simulink model "Tank_test_init_sim_2017b"  (R2017b)
settings: Solver=FixedStepAuto  StartTime=0.0  StopTime=Endtime  FixedStep=Ts_sys  RelTol=1e-3
StopFcn:
  | %ファイル出力
  | %======================== 全体 =================================
  | time = Tank_IOdata_All.time;
  | %状態変数
  | Pipe_Temp1 = Tank_IOdata_All.signals.values(:, 1);
  | Pipe_Temp2 = Tank_IOdata_All.signals.values(:, 2);
  | Pipe_Temp3 = Tank_IOdata_All.signals.values(:, 3);
  | Tank1_Height = Tank_IOdata_All.signals.values(:, 4);
  | Tank2_Height = Tank_IOdata_All.signals.values(:, 5);
  | Cold_Flow = Tank_IOdata_All.signals.values(:, 6);
  | Hot_Flow = Tank_IOdata_All.signals.values(:, 7);
  | Discharge_Flow1 =  Tank_IOdata_All.signals.values(:, 8);
  | Discharge_Flow2 =  Tank_IOdata_All.signals.values(:, 9);
  | %入力
  | u_Cold =  Tank_IOdata_All.signals.values(:, 10);
  | u_Hot =  Tank_IOdata_All.signals.values(:, 11);
  | u_Heater =  Tank_IOdata_All.signals.values(:, 12);
  | u_Valve =  Tank_IOdata_All.signals.values(:, 13);
  | 
  | %ファイル出力
  | filename = 'Tank_test';
  | %matファイル出力
  | save([filename, '.mat']);
  | %csv出力
  | fid = fopen([filename, '.csv'],'w');
  | fprintf(fid, ['%%time[s], Pipe_Temp1[deg], Pipe_Temp2[deg], Pipe_Temp3[deg], Tank1_Height[mm], Tank2_Height[mm], Cold_Flow[L/min], Hot_Flow[L/min], Discharge_Flow1[L/min], Discharge_Flow2[L/min], u_Cold[%%], u_Hot[%%], u_Heater[%%], u_Valve[%%]\n']);
  | fprintf(fid, ['%f, %f, %f, %f, %f, %f, %f, %f, %f, %f, %f, %f, %f, %f\n'], [time, Tank_IOdata_All.signals.values]');
  | fclose(fid);
  | %======================== 全体 =================================
values from neighbouring files (symbols this model uses):
  Tank_IOdata_All =     [Tank_test.mat]
  Ts = 1    [Tank_test.m]    (also in Tank_test.mat; dd_frit_pid_sim.m; frit_pid.m)
undefined symbols (not defined in the file or in its folder): National_Instruments, PCIe
libraries: sldrtlib x14, simulink x1
settings Model: Creator=CSELab  LastModifiedBy=CSELab
settings OptimizationCC: EfficientMapNaN2IntZero=off
settings HardwareCC: TargetBitPerPointer=64  TargetBitPerSizeT=64  TargetBitPerPtrDiffT=64  TargetLongLongMode=on  TargetIntDivRoundTo=Zero  TargetEndianess=LittleEndian  TargetWordSize=64  TargetHWDeviceType=MATLAB Host  ProdEqTarget=off
settings CodeAppCC: MaxIdLength=128
settings GRTTargetCC: TargetLangStandard=C89/C90 (ANSI)  CombineOutputUpdateFcns=off  GRTInterface=on

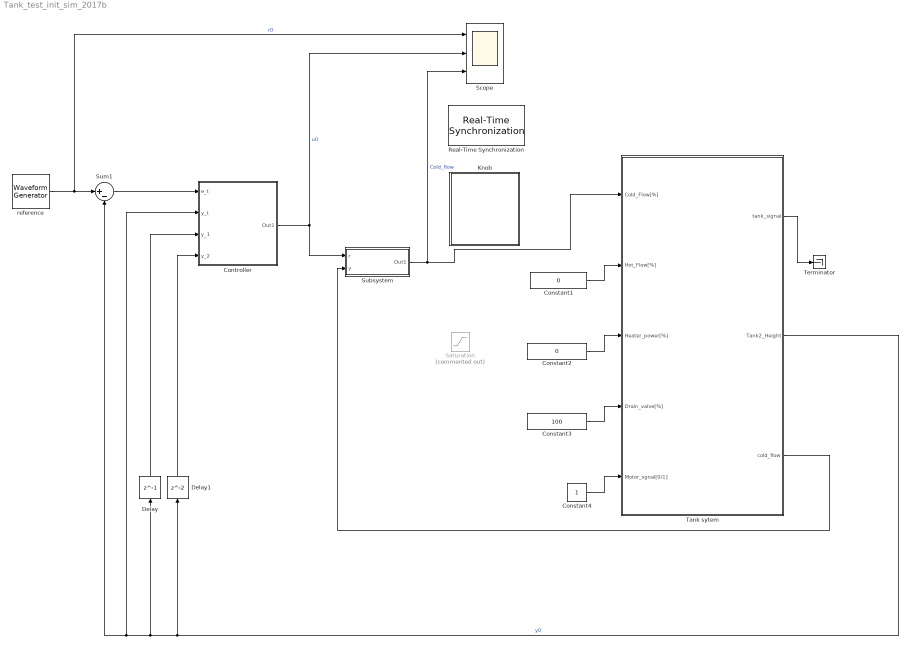
== system Tank_test_init_sim_2017b ==
  Constant1 : Constant  Value=0
  Constant2 : Constant  Value=0
  Constant3 : Constant  Value=100
  Constant4 : Constant
  "Controller " : Subsystem
  Delay : Delay  DelayLength=1  SampleTime=Ts
  Delay1 : Delay  SampleTime=Ts
  Knob : Subsystem  DialogController=hmiCreateDDGDialog  IsWebBlock=on  mask(MWDashboardBlock){webBlockId=6c2fbc2a-5fc2-4e4f-923f-305dcc113598, webBlockType=continuousknob, ShowInLibBrowser=on, ShowInitialText=on, HMISrcModelName=Tank_test_init_sim_2017b}
      mask prompts: webBlockId "WebBlock Id"; webBlockType "WebBlock Type"; HMISrcModelName "Source Model"
      mask help: Set a value to tune parameters or variables.
      mask Help: helpview([docroot '/mapfiles/simulink.map'], 'hmi_knob')
      mask Display:
      | if strcmp(get_param(bdroot(gcb),'BlockDiagramType'),'library')
      |  image([(matlabroot) '/toolbox/simulink/hmi/icons/ContinuousKnob.png'])
      | end
  Real-Time Synchronization : sldrtlib/Real-Time Synchronization  SampleTime=-1  MaxMissedTicks=10  ShowMissedTicks=off  YieldWhenWaiting=off
  Saturation : Saturate  Commented=on  UpperLimit=100  LowerLimit=0
  Scope : Scope  NumInputPorts=3
  Subsystem : Subsystem
  Sum1 : Sum  Inputs=|+-
  Tank sytem : Subsystem
  Terminator : Terminator
  "reference " : simulink/Sources/Waveform Generator  OutMin=[]  OutMax=[]  OutDataTypeStr=double  SelectedSignal=1  Signals=step(0,0,100) + step(350,0,50)  BlockNames=MultiportSwitch_95f7518ff940498  SampleTime=Ts
      settings: SourceProductName=Simulink
  wires:
  Constant1/1 -> Tank sytem/2(Hot_Flow[%])
  Constant2/1 -> Tank sytem/3(Heater_power[%])
  Constant3/1 -> Tank sytem/4(Drain_valve[%])
  Tank sytem/1(tank_signal) -> Terminator/1
  Constant4/1 -> Tank sytem/5(Motor_sgnal[0/1])
  Delay1/1 -> "Controller "/4(y_2)
  Delay/1 -> "Controller "/3("y_1 ")
  Tank sytem/2(Tank2_Height) -> Delay1/1, Sum1/2, "Controller "/2(y_t), Delay/1  "y0"
  "Controller "/1(Out1) -> Scope/2, Subsystem/1(r)  "u0"
  "reference "/1 -> Scope/1, Sum1/1  "r0"
  Sum1/1 -> "Controller "/1("e_t ")
  Tank sytem/3("cold_flow ") -> Subsystem/2(y)
  Subsystem/1(Out1) -> Tank sytem/1(Cold_Flow[%]), Scope/3  "Cold_flow"

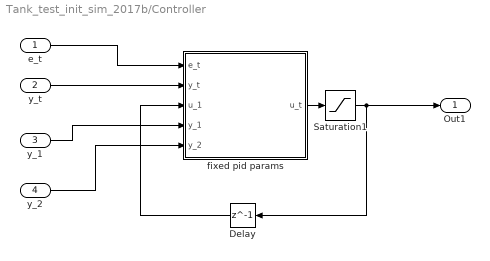
== system Tank_test_init_sim_2017b/Controller  ==
  "e_t " : Inport
  y_t : Inport  Port=2
  "y_1 " : Inport  Port=3
  y_2 : Inport  Port=4
  Delay : Delay  DelayLength=1  SampleTime=Ts
  Saturation1 : Saturate  UpperLimit=40  LowerLimit=10
  fixed pid params : MATLAB Function  TreatAsAtomicUnit=on
  Out1 : Outport
  wires:
  "e_t "/1 -> fixed pid params/1(e_t)
  fixed pid params/1(u_t) -> Saturation1/1
  Delay/1 -> fixed pid params/3(u_1)
  "y_1 "/1 -> fixed pid params/4(y_1)
  y_2/1 -> fixed pid params/5(y_2)
  y_t/1 -> fixed pid params/2(y_t)
  Saturation1/1 -> Delay/1, Out1/1

== system Tank_test_init_sim_2017b/Knob ==

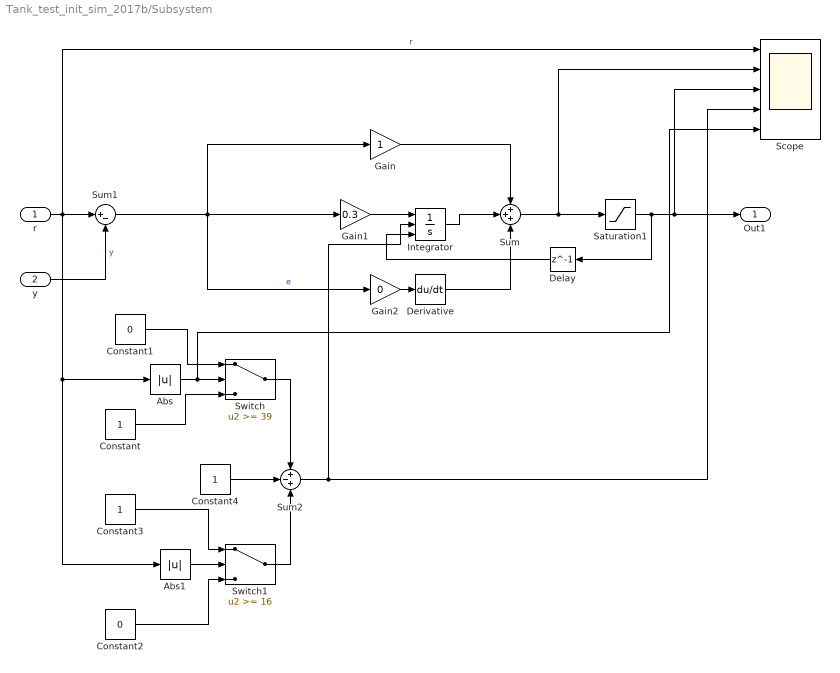
== system Tank_test_init_sim_2017b/Subsystem ==
  r : Inport
  y : Inport  Port=2
  Abs : Abs
  Abs1 : Abs
  Constant : Constant
  Constant1 : Constant  Value=0
  Constant2 : Constant  Value=0
  Constant3 : Constant
  Constant4 : Constant
  Delay : Delay  DelayLength=1  SampleTime=Ts
  Derivative : Derivative
  Gain : Gain
  Gain1 : Gain  Gain=0.3
  Gain2 : Gain  Gain=0
  Integrator : Integrator  ExternalReset=rising  InitialConditionSource=external
  Saturation1 : Saturate  UpperLimit=40  LowerLimit=0
  Scope : Scope  NumInputPorts=5
  Sum : Sum  Inputs=+++
  Sum1 : Sum  Inputs=|+-
  Sum2 : Sum  Inputs=+-+
  Switch : Switch  Threshold=39
  Switch1 : Switch  Threshold=16
  Out1 : Outport
  wires:
  Derivative/1 -> Sum/3
  r/1 -> Abs1/1, Abs/1, Scope/1, Sum1/1  "r"
  Sum1/1 -> Gain2/1, Gain/1, Gain1/1  "e"
  y/1 -> Sum1/2  "y"
  Gain1/1 -> Integrator/1
  Saturation1/1 -> Delay/1, Scope/3, Out1/1
  Gain2/1 -> Derivative/1
  Gain/1 -> Sum/1
  Sum/1 -> Scope/2, Saturation1/1
  Integrator/1 -> Sum/2
  Constant/1 -> Switch/3
  Constant1/1 -> Switch/1
  Switch/1 -> Sum2/1
  Abs/1 -> Scope/5, Switch/2
  Abs1/1 -> Switch1/2
  Constant2/1 -> Switch1/3
  Constant3/1 -> Switch1/1
  Sum2/1 -> Scope/4, Integrator/2
  Switch1/1 -> Sum2/3
  Constant4/1 -> Sum2/2
  Delay/1 -> Integrator/3

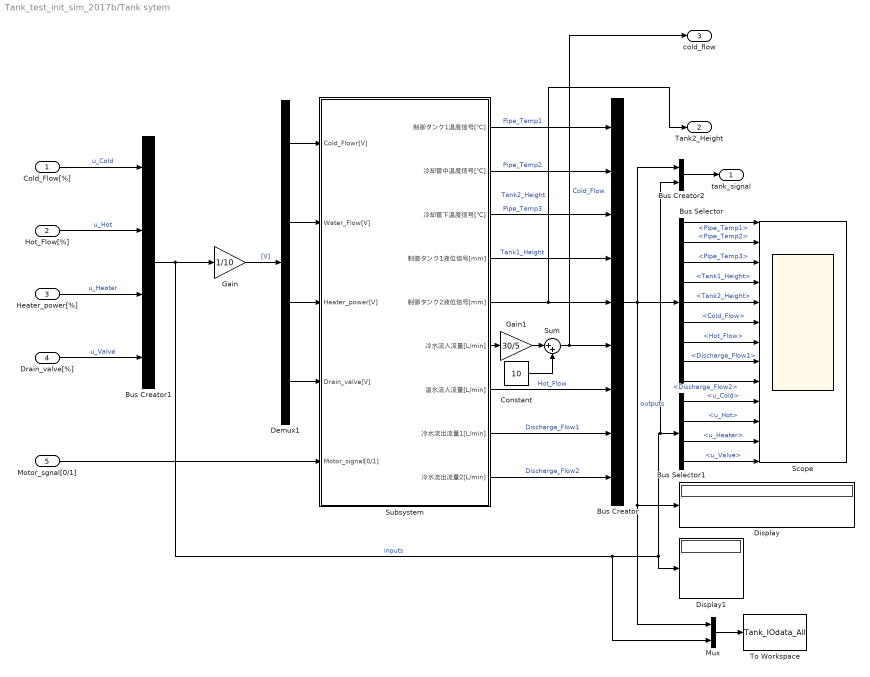
== system Tank_test_init_sim_2017b/Tank sytem ==
  Cold_Flow[%] : Inport
  Hot_Flow[%] : Inport  Port=2
  Heater_power[%] : Inport  Port=3
  Drain_valve[%] : Inport  Port=4
  Motor_sgnal[0/1] : Inport  Port=5
  Bus Creator : BusCreator  Inputs=9
  Bus Creator1 : BusCreator  Inputs=4
  Bus Creator2 : BusCreator  Inputs=2
  Bus Selector : BusSelector  OutputSignals=Pipe_Temp1,Pipe_Temp2,Pipe_Temp3,Tank1_Height,Tank2_Height,Cold_Flow,Hot_Flow,Discharge_Flow1,Discharge_Flow2
  Bus Selector1 : BusSelector  OutputSignals=u_Cold,u_Hot,u_Heater,u_Valve
  Constant : Constant  Value=10
  Demux1 : Demux
  Display : Display
  Display1 : Display
  Gain : Gain  Gain=1/10
  Gain1 : Gain  Gain=30/5
  Mux : Mux  Inputs=2
  Scope : Scope  NumInputPorts=13
  Subsystem : Subsystem
  Sum : Sum  Inputs=|++
  To Workspace : ToWorkspace  VariableName=Tank_IOdata_All  SaveFormat=Structure With Time  SampleTime=-1
  tank_signal : Outport
  Tank2_Height : Outport  Port=2
  "cold_flow " : Outport  Port=3
  wires:
  Heater_power[%]/1 -> Bus Creator1/3  "u_Heater"
  Bus Creator1/1 -> Gain/1, Mux/2, Display1/1, Bus Creator2/2, Bus Selector1/1  "inputs"
  Hot_Flow[%]/1 -> Bus Creator1/2  "u_Hot"
  Cold_Flow[%]/1 -> Bus Creator1/1  "u_Cold"
  Subsystem/1(制御タンク1温度信号[℃]) -> Bus Creator/1  "Pipe_Temp1"
  Subsystem/2(冷却管中温度信号[℃]) -> Bus Creator/2  "Pipe_Temp2"
  Subsystem/5(制御タンク2液位信号[mm]) -> Tank2_Height/1, Bus Creator/5  "Tank2_Height"
  Demux1/3 -> Subsystem/3(Heater_power[V])
  Demux1/1 -> Subsystem/1(Cold_Flowr[V])
  Demux1/2 -> Subsystem/2(Water_Flow[V])
  Subsystem/4(制御タンク1液位信号[mm]) -> Bus Creator/4  "Tank1_Height"
  Subsystem/3(冷却管下温度信号[℃]) -> Bus Creator/3  "Pipe_Temp3"
  Drain_valve[%]/1 -> Bus Creator1/4  "u_Valve"
  Demux1/4 -> Subsystem/4(Drain_valve[V])
  Gain/1 -> Demux1/1  "[V]"
  Subsystem/7(温水流入流量[L/min]) -> Bus Creator/7  "Hot_Flow"
  Subsystem/8(冷水流出流量1[L/min]) -> Bus Creator/8  "Discharge_Flow1"
  Subsystem/9(冷水流出流量2[L/min]) -> Bus Creator/9  "Discharge_Flow2"
  Bus Creator/1 -> Bus Creator2/1, Bus Selector/1, Mux/1, Display/1  "outputs"
  Bus Selector/1 -> Scope/1  "<Pipe_Temp1>"
  Bus Selector/2 -> Scope/2  "<Pipe_Temp2>"
  Bus Selector/3 -> Scope/3  "<Pipe_Temp3>"
  Bus Selector/4 -> Scope/4  "<Tank1_Height>"
  Bus Selector/5 -> Scope/5  "<Tank2_Height>"
  Bus Selector/6 -> Scope/6  "<Cold_Flow>"
  Bus Selector/7 -> Scope/7  "<Hot_Flow>"
  Bus Selector/8 -> Scope/8  "<Discharge_Flow1>"
  Bus Selector/9 -> Scope/9  "<Discharge_Flow2>"
  Bus Selector1/1 -> Scope/10  "<u_Cold>"
  Bus Selector1/2 -> Scope/11  "<u_Hot>"
  Bus Selector1/3 -> Scope/12  "<u_Heater>"
  Bus Selector1/4 -> Scope/13  "<u_Valve>"
  Mux/1 -> To Workspace/1
  Bus Creator2/1 -> tank_signal/1
  Motor_sgnal[0/1]/1 -> Subsystem/5(Motor_signal[0/1])
  Subsystem/6(冷水流入流量[L/min]) -> Gain1/1
  Gain1/1 -> Sum/1
  Constant/1 -> Sum/2
  Sum/1 -> Bus Creator/6, "cold_flow "/1  "Cold_Flow"

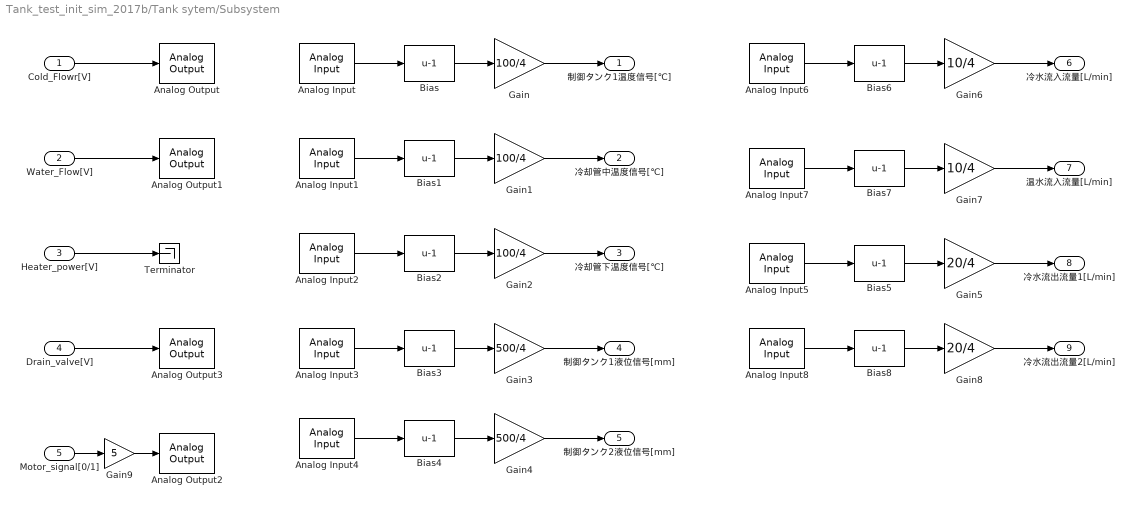
== system Tank_test_init_sim_2017b/Tank sytem/Subsystem ==
  Cold_Flowr[V] : Inport
  Water_Flow[V] : Inport  Port=2
  Heater_power[V] : Inport  Port=3
  Drain_valve[V] : Inport  Port=4
  Motor_signal[0/1] : Inport  Port=5
  Analog Input : sldrtlib/Analog Input  SampleTime=-1  MaxMissedTicks=10  ShowMissedTicks=off  YieldWhenWaiting=off  DrvName=National_Instruments/PCIe-6323  DrvAddress=4294967295  DrvOptions=[0 0 0 0 0 0 0]  Channels=1  RangeMode=1  VoltRange=1  DataType=1
      settings: AttributesFormatString=National Instruments\nPCIe-6323 [auto]  SourceProductName=Simulink Desktop Real-Time
  Analog Input1 : sldrtlib/Analog Input  SampleTime=-1  MaxMissedTicks=10  ShowMissedTicks=off  YieldWhenWaiting=off  DrvName=National_Instruments/PCIe-6323  DrvAddress=4294967295  DrvOptions=[0 0 0 0 0 0 0]  Channels=2  RangeMode=1  VoltRange=1  DataType=1
      settings: AttributesFormatString=National Instruments\nPCIe-6323 [auto]  SourceProductName=Simulink Desktop Real-Time
  Analog Input2 : sldrtlib/Analog Input  SampleTime=-1  MaxMissedTicks=10  ShowMissedTicks=off  YieldWhenWaiting=off  DrvName=National_Instruments/PCIe-6323  DrvAddress=4294967295  DrvOptions=[0 0 0 0 0 0 0]  Channels=3  RangeMode=1  VoltRange=1  DataType=1
      settings: AttributesFormatString=National Instruments\nPCIe-6323 [auto]  SourceProductName=Simulink Desktop Real-Time
  Analog Input3 : sldrtlib/Analog Input  SampleTime=-1  MaxMissedTicks=10  ShowMissedTicks=off  YieldWhenWaiting=off  DrvName=National_Instruments/PCIe-6323  DrvAddress=4294967295  DrvOptions=[0 0 0 0 0 0 0]  Channels=4  RangeMode=1  VoltRange=1  DataType=1
      settings: AttributesFormatString=National Instruments\nPCIe-6323 [auto]  SourceProductName=Simulink Desktop Real-Time
  Analog Input4 : sldrtlib/Analog Input  SampleTime=-1  MaxMissedTicks=10  ShowMissedTicks=off  YieldWhenWaiting=off  DrvName=National_Instruments/PCIe-6323  DrvAddress=4294967295  DrvOptions=[0 0 0 0 0 0 0]  Channels=5  RangeMode=1  VoltRange=1  DataType=1
      settings: AttributesFormatString=National Instruments\nPCIe-6323 [auto]  SourceProductName=Simulink Desktop Real-Time
  Analog Input5 : sldrtlib/Analog Input  SampleTime=-1  MaxMissedTicks=10  ShowMissedTicks=off  YieldWhenWaiting=off  DrvName=National_Instruments/PCIe-6323  DrvAddress=4294967295  DrvOptions=[0 0 0 0 0 0 0]  Channels=9  RangeMode=1  VoltRange=1  DataType=1
      settings: AttributesFormatString=National Instruments\nPCIe-6323 [auto]  SourceProductName=Simulink Desktop Real-Time
  Analog Input6 : sldrtlib/Analog Input  SampleTime=-1  MaxMissedTicks=10  ShowMissedTicks=off  YieldWhenWaiting=off  DrvName=National_Instruments/PCIe-6323  DrvAddress=4294967295  DrvOptions=[0 0 0 0 0 0 0]  Channels=7  RangeMode=1  VoltRange=1  DataType=1
      settings: AttributesFormatString=National Instruments\nPCIe-6323 [auto]  SourceProductName=Simulink Desktop Real-Time
  Analog Input7 : sldrtlib/Analog Input  SampleTime=-1  MaxMissedTicks=10  ShowMissedTicks=off  YieldWhenWaiting=off  DrvName=National_Instruments/PCIe-6323  DrvAddress=4294967295  DrvOptions=[0 0 0 0 0 0 0]  Channels=8  RangeMode=1  VoltRange=1  DataType=1
      settings: AttributesFormatString=National Instruments\nPCIe-6323 [auto]  SourceProductName=Simulink Desktop Real-Time
  Analog Input8 : sldrtlib/Analog Input  SampleTime=-1  MaxMissedTicks=10  ShowMissedTicks=off  YieldWhenWaiting=off  DrvName=National_Instruments/PCIe-6323  DrvAddress=4294967295  DrvOptions=[0 0 0 0 0 0 0]  Channels=10  RangeMode=1  VoltRange=1  DataType=1
      settings: AttributesFormatString=National Instruments\nPCIe-6323 [auto]  SourceProductName=Simulink Desktop Real-Time
  Analog Output : sldrtlib/Analog Output  SampleTime=-1  MaxMissedTicks=10  ShowMissedTicks=off  YieldWhenWaiting=off  DrvName=National_Instruments/PCIe-6323  DrvAddress=4294967295  DrvOptions=[0 0 0 0 0 0 0]  Channels=1  RangeMode=1  VoltRange=1  InitialValue=0  FinalValue=0
      settings: AttributesFormatString=National Instruments\nPCIe-6323 [auto]  SourceProductName=Simulink Desktop Real-Time
  Analog Output1 : sldrtlib/Analog Output  SampleTime=-1  MaxMissedTicks=10  ShowMissedTicks=off  YieldWhenWaiting=off  DrvName=National_Instruments/PCIe-6323  DrvAddress=4294967295  DrvOptions=[0 0 0 0 0 0 0]  Channels=2  RangeMode=1  VoltRange=1  InitialValue=0  FinalValue=0
      settings: AttributesFormatString=National Instruments\nPCIe-6323 [auto]  SourceProductName=Simulink Desktop Real-Time
  Analog Output2 : sldrtlib/Analog Output  SampleTime=-1  MaxMissedTicks=10  ShowMissedTicks=off  YieldWhenWaiting=off  DrvName=National_Instruments/PCIe-6323  DrvAddress=4294967295  DrvOptions=[0 0 0 0 0 0 0]  Channels=3  RangeMode=1  VoltRange=1  InitialValue=0  FinalValue=0
      settings: AttributesFormatString=National Instruments\nPCIe-6323 [auto]  SourceProductName=Simulink Desktop Real-Time
  Analog Output3 : sldrtlib/Analog Output  SampleTime=-1  MaxMissedTicks=10  ShowMissedTicks=off  YieldWhenWaiting=off  DrvName=National_Instruments/PCIe-6323  DrvAddress=4294967295  DrvOptions=[0 0 0 0 0 0 0]  Channels=4  RangeMode=1  VoltRange=1  InitialValue=0  FinalValue=10
      settings: AttributesFormatString=National Instruments\nPCIe-6323 [auto]  SourceProductName=Simulink Desktop Real-Time
  Bias{,1..8} (9 alike) : Bias  Bias=-1
  Gain : Gain  Gain=100/4
  Gain1 : Gain  Gain=100/4
  Gain2 : Gain  Gain=100/4
  Gain3 : Gain  Gain=500/4
  Gain4 : Gain  Gain=500/4
  Gain5 : Gain  Gain=20/4
  Gain6 : Gain  Gain=10/4
  Gain7 : Gain  Gain=10/4
  Gain8 : Gain  Gain=20/4
  Gain9 : Gain  Gain=5
  Terminator : Terminator
  制御タンク1温度信号[℃] : Outport
  冷却管中温度信号[℃] : Outport  Port=2
  冷却管下温度信号[℃] : Outport  Port=3
  制御タンク1液位信号[mm] : Outport  Port=4
  制御タンク2液位信号[mm] : Outport  Port=5
  冷水流入流量[L/min] : Outport  Port=6
  温水流入流量[L/min] : Outport  Port=7
  冷水流出流量1[L/min] : Outport  Port=8
  冷水流出流量2[L/min] : Outport  Port=9
  wires:
  Bias/1 -> Gain/1
  Water_Flow[V]/1 -> Analog Output1/1
  Analog Input/1 -> Bias/1
  Analog Input1/1 -> Bias1/1
  Analog Input4/1 -> Bias4/1
  Analog Input2/1 -> Bias2/1
  Analog Input3/1 -> Bias3/1
  Gain1/1 -> 冷却管中温度信号[℃]/1
  Gain2/1 -> 冷却管下温度信号[℃]/1
  Bias2/1 -> Gain2/1
  Bias1/1 -> Gain1/1
  Bias4/1 -> Gain4/1
  Gain4/1 -> 制御タンク2液位信号[mm]/1
  Gain3/1 -> 制御タンク1液位信号[mm]/1
  Bias3/1 -> Gain3/1
  Gain/1 -> 制御タンク1温度信号[℃]/1
  Heater_power[V]/1 -> Terminator/1
  Cold_Flowr[V]/1 -> Analog Output/1
  Analog Input5/1 -> Bias5/1
  Bias5/1 -> Gain5/1
  Analog Input6/1 -> Bias6/1
  Gain6/1 -> 冷水流入流量[L/min]/1
  Bias6/1 -> Gain6/1
  Bias7/1 -> Gain7/1
  Analog Input7/1 -> Bias7/1
  Gain7/1 -> 温水流入流量[L/min]/1
  Gain8/1 -> 冷水流出流量2[L/min]/1
  Analog Input8/1 -> Bias8/1
  Bias8/1 -> Gain8/1
  Drain_valve[V]/1 -> Analog Output3/1
  Gain5/1 -> 冷水流出流量1[L/min]/1
  Motor_signal[0/1]/1 -> Gain9/1
  Gain9/1 -> Analog Output2/1

== matlab function Tank_test_init_sim_2017b/Controller /fixed pid params ==
  data: e_t input; u_t output; y_t input; u_1 input; y_1 input; y_2 input; K parameter
function u_t = fcn(e_t, y_t, u_1, y_1, y_2, K)

u_t = u_1 + K(2)*(e_t) - K(1)*(y_t - y_1) - K(3)*(y_t - 2*y_1 + y_2);
